simulink model "inverse_position_model"  (R2020a)
settings: Solver=VariableStepAuto  StartTime=0.0  StopTime=10.0  RelTol=1e-3
settings Model: Creator=Lord  LastModifiedBy=Lord

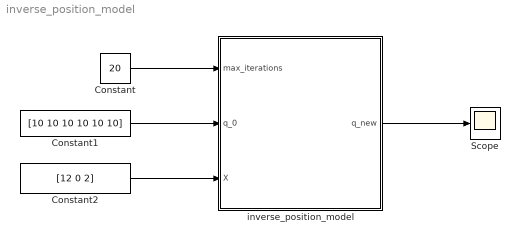
== system inverse_position_model ==
  Constant : Constant  Value=20
  Constant1 : Constant  Value=[10 10 10 10 10 10]
  Constant2 : Constant  Value=[12 0 2]
  Scope : Scope
  inverse_position_model : MATLAB Function  TreatAsAtomicUnit=on
  wires:
  Constant1/1 -> inverse_position_model/2(q_0)
  Constant/1 -> inverse_position_model/1(max_iterations)
  Constant2/1 -> inverse_position_model/3(X)
  inverse_position_model/1(q_new) -> Scope/1

== matlab function inverse_position_model/inverse_position_model ==
  data: max_iterations input; q_new output; q_0 input; X input
function  q_new = inverse_position_model(max_iterations,q_0,X)
i=0;
q_new = zeros(6,1)
q_00=q_0;
while i< max_iterations
    j_inv=inverse_jacobian_matrix(q_00);
    [tt,qq] = end_effec_num(q_00);
    q_new=transpose(q_00)-(j_inv)*(transpose(qq)-X);
    for i=1:6
        if(q_new(i,1)>360 | q_new(i,1)<-360 )
            q_new(i,1)=mod(q_new(i,1),360);
        end
    end

    q_00=transpose(q_new);
    i=i+1;
end
end
